simulink model "Phase_Lead_sim"  (R2023b)
settings: Solver=VariableStepAuto  StartTime=0.0  StopTime=10.0  RelTol=1e-3
libraries: cstblocks x4, simulink x1
settings Model: Creator=elias  LastModifiedBy=elias

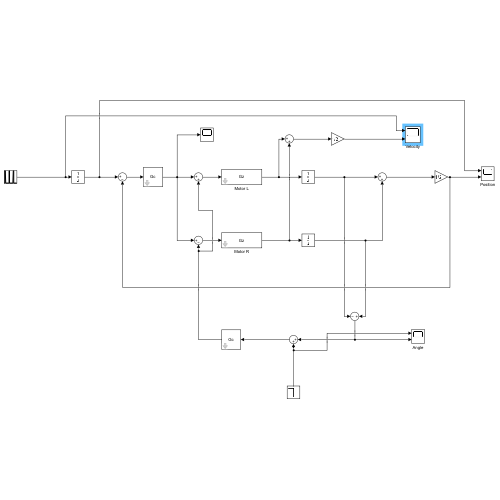
[thumbnail: Simulink's stored preview of the top-level diagram]
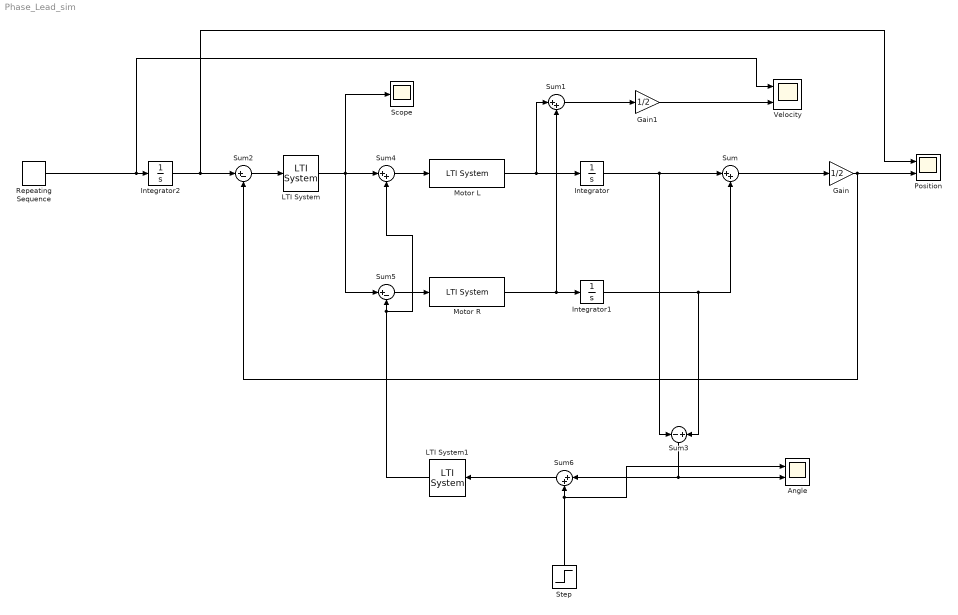
== system Phase_Lead_sim ==
  Angle : Scope  NumInputPorts=2
  Gain : Gain  Gain=1/2
  Gain1 : Gain  Gain=1/2
  Integrator : Integrator
  Integrator1 : Integrator
  Integrator2 : Integrator
  LTI System : cstblocks/LTI System  sys=Gc  IC=[]  PadeOrder=0
  LTI System1 : cstblocks/LTI System  sys=Gc  IC=[]  PadeOrder=0
  Motor L : cstblocks/LTI System  sys=Gz  IC=[]  PadeOrder=0
  Motor R : cstblocks/LTI System  sys=Gz  IC=[]  PadeOrder=0
  Position : Scope  NumInputPorts=2
  Repeating Sequence : simulink/Sources/Repeating Sequence  rep_seq_t=[0 2 2.5 5 5.5 20]  rep_seq_y=[0 0 250 250 0 0]
  Scope : Scope
  Step : Step  After=-90  SampleTime=0
  Sum{,1,4,6} (4 alike) : Sum  Inputs=|++
  Sum2 : Sum  Inputs=|+-
  Sum3 : Sum  Inputs=-+
  Sum5 : Sum  Inputs=|+-
  Velocity : Scope  NumInputPorts=2
  wires:
  Sum5/1 -> Motor R/1
  Motor R/1 -> Sum1/2, Integrator1/1
  Sum4/1 -> Motor L/1
  Sum3/1 -> Angle/2, Sum6/1
  LTI System1/1 -> Sum4/2, Sum5/2
  Step/1 -> Angle/1, Sum6/2
  Gain1/1 -> Velocity/2
  Sum1/1 -> Gain1/1
  Integrator2/1 -> Sum2/1, Position/1
  Gain/1 -> Sum2/2, Position/2
  Sum/1 -> Gain/1
  Integrator/1 -> Sum3/1, Sum/1
  Integrator1/1 -> Sum3/2, Sum/2
  Repeating Sequence/1 -> Velocity/1, Integrator2/1
  Sum6/1 -> LTI System1/1
  LTI System/1 -> Sum4/1, Scope/1, Sum5/1
  Motor L/1 -> Sum1/1, Integrator/1
  Sum2/1 -> LTI System/1
